simulink model "vloop_test_modify2017"  (R2017a)
settings: Solver=FixedStepAuto  StartTime=0.0  StopTime=Tf  FixedStep=delta_r  RelTol=1e-3  EnableMultiTasking=on
InitFcn:
  | G = 107.815;
values from neighbouring files (symbols this model uses):
  delta_r = 1/1000    (= 0.001)    [p560_simulation_main_velocity2017.m]
  delta_t = 1/200    (= 0.005)    [p560_simulation_main_velocity2017.m]
  Kd = 0.0006    [p560_simulation_main_velocity2017.m]
  time_delay = 0    [p560_simulation_main_velocity2017.m]
undefined symbols (not defined in the file or in its folder): yh
libraries: sldrtlib x1, simulink x1
Description:
  | vloop parameters for
  | Puma560 shoulder joint
  | with link inertia
  | RVC1 p.205
settings Model: DisableUpgradeWarningsForVersion=R2014b  Creator=pic  LastModifiedBy=yehanspc
settings DataIOCC: LimitDataPoints=on  SaveFormat=Array  SignalLoggingSaveFormat=ModelDataLogs  ReturnWorkspaceOutputs=on  TimeSaveName=t  OutputSaveName=y
settings OptimizationCC: ExpressionDepthLimit=2147483647  LifeSpan=inf
settings DebuggingCC: UnderspecifiedInitializationDetection=Classic  MergeDetectMultiDrivingBlocksExec=none  SolverPrmCheckMsg=warning  MultiTaskRateTransMsg=warning  FcnCallInpInsideContextMsg=warning  AllowSymbolicDim=off  StateNameClashWarn=warning  SFUnexpectedBacktrackingDiag=warning  SFNoUnconditionalDefaultTransitionDiag=warning  SFExecutionAtInitializationDiag=none
settings HardwareCC: ProdBitPerPointer=32  ProdBitPerSizeT=32  ProdBitPerPtrDiffT=32  ProdLargestAtomicFloat=None  ProdIntDivRoundTo=Undefined  ProdEndianess=Unspecified  ProdWordSize=32  ProdHWDeviceType=32-bit Generic
settings ModelReferenceCC: PropagateSignalLabelsOutOfModel=off
settings SFSimCC: SimCustomInitializer=|
  | if ~exist(tau_d)
  |    tau_d = 0
  | end
settings GRTTargetCC: TargetLangStandard=C89/C90 (ANSI)  GeneratePreprocessorConditionals=Disable all  CombineOutputUpdateFcns=off  GRTInterface=on
settings ConfigComp: CovMetricSettings=dw  CovHtmlReporting=on  CovSaveCumulativeToWorkspaceVar=on  CovSaveSingleToWorkspaceVar=on  CovExternalEMLEnable=off  CovSFcnEnable=off

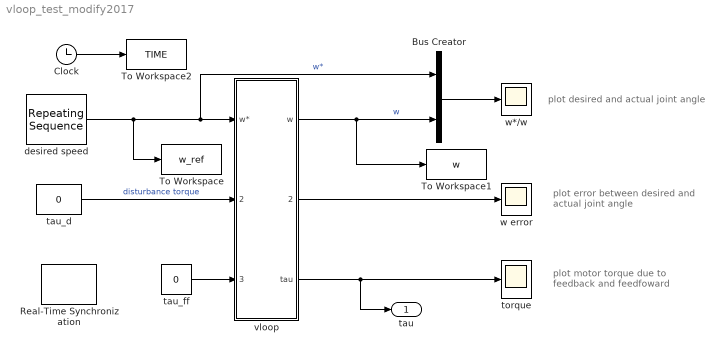
== system vloop_test_modify2017 ==
  note: plot motor torque due
      | to feedback and feedfoward
  note: plot error between desired and
      | actual joint angle
  note: plot desired and actual joint angle
  Bus Creator : BusCreator  Inputs=2
  Clock : Clock
  Real-Time Synchronization : sldrtlib/Real-Time Synchronization  SampleTime=delta_t  MaxMissedTicks=10000  ShowMissedTicks=off  YieldWhenWaiting=off
  To Workspace : ToWorkspace  VariableName=w_ref  SaveFormat=Timeseries  SampleTime=-1
  To Workspace1 : ToWorkspace  VariableName=w  SaveFormat=Timeseries  SampleTime=-1
  To Workspace2 : ToWorkspace  VariableName=TIME  SaveFormat=Timeseries  SampleTime=-1
  desired speed : simulink/Sources/Repeating Sequence  rep_seq_t=[0 1 3 4 6]/10  rep_seq_y=[50 50 50 50 50]
  tau_d : Constant  Value=0
  tau_ff : Constant  Value=0
  torque : Scope
  vloop : Subsystem  AncestorBlock=roblocks/Arm/vloop  mask{J=580e-6, B=817e-6, Km=0.228, tau_max=0.9, Kv=0.3, Ki=0.2, T=0.001}
      mask prompts: J "Inertia (J)"; B "Viscous friction coefficient (B)"; Km "Motor torque constant"; tau_max "Torque limit (tau_max)"; Kv "Proportional gain (Kv)"; Ki "Integral gain (Ki)"; T "Sample interval (T)"
  w error : Scope
  w*/w : Scope
  tau : Outport
  wires:
  desired speed/1 -> To Workspace/1, Bus Creator/1, vloop/1(w*)  "w*"
  Bus Creator/1 -> w*/w/1
  vloop/1(w) -> To Workspace1/1, Bus Creator/2  "w"
  vloop/2(w error) -> w error/1
  vloop/3(tau) -> torque/1, tau/1
  tau_d/1 -> vloop/2(tau_d)  "disturbance torque"
  tau_ff/1 -> vloop/3(tau_ff)
  Clock/1 -> To Workspace2/1

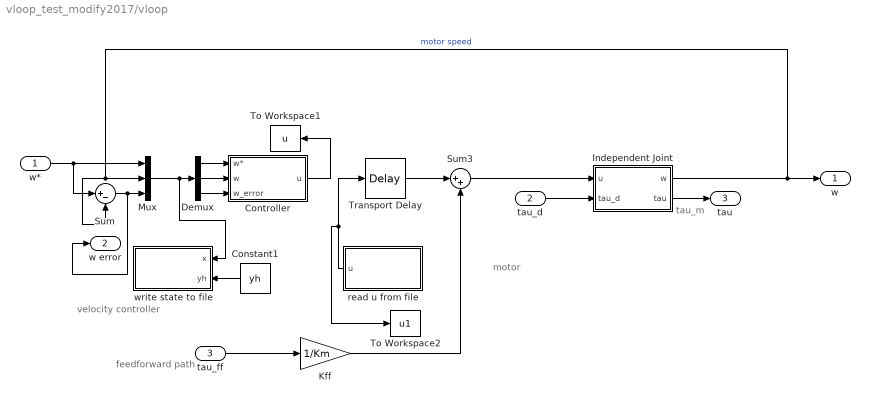
== system vloop_test_modify2017/vloop ==
  note: velocity controller
  note: feedforward path
  note: tau_m
  note: motor
  w* : Inport
  tau_d : Inport  Port=2
  tau_ff : Inport  Port=3
  Constant1 : Constant  Value=yh
  Controller : Subsystem
  Demux : Demux  Outputs=3
  Independent Joint : Subsystem
  Kff : Gain  Gain=1/Km
  Mux : Mux  Inputs=3
  Sum : Sum  Inputs=|+-
  Sum3 : Sum  Inputs=|++
  To Workspace1 : ToWorkspace  VariableName=u  SaveFormat=Timeseries  SampleTime=-1
  To Workspace2 : ToWorkspace  VariableName=u1  SaveFormat=Timeseries  SampleTime=-1
  Transport Delay : TransportDelay  DelayTime=time_delay
  read u from file : MATLAB Function  TreatAsAtomicUnit=on
  write state to file : MATLAB Function  TreatAsAtomicUnit=on
  w : Outport
  w error : Outport  Port=2
  tau : Outport  Port=3
  wires:
  tau_ff/1 -> Kff/1
  Kff/1 -> Sum3/2
  Sum3/1 -> Independent Joint/1(u)
  tau_d/1 -> Independent Joint/2(tau_d)
  Independent Joint/1(w) -> Mux/2, Sum/2, w/1  "motor speed"
  w*/1 -> Mux/1, Sum/1
  Sum/1 -> Mux/3, w error/1
  Transport Delay/1 -> Sum3/1
  Independent Joint/2(tau) -> tau/1
  Mux/1 -> Demux/1, write state to file/1(x)
  Constant1/1 -> write state to file/2(yh)
  Demux/1 -> Controller/1(w*)
  Demux/2 -> Controller/2(w)
  Demux/3 -> Controller/3(w_error)
  Controller/1(u) -> To Workspace1/1
  read u from file/1(u) -> To Workspace2/1, Transport Delay/1

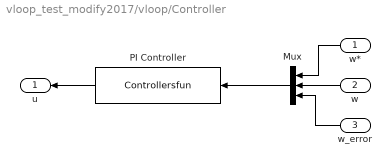
== system vloop_test_modify2017/vloop/Controller ==
  w* : Inport
  w : Inport  Port=2
  w_error : Inport  Port=3
  Mux : Mux  Inputs=3
  PI Controller : S-Function  FunctionName=Controllersfun  Parameters=Kv,Ki,Kd,delta_t,delta_r  SFunctionDeploymentMode=off  EnableBusSupport=off
  u : Outport
  wires:
  w/1 -> Mux/2
  w*/1 -> Mux/1
  Mux/1 -> PI Controller/1
  PI Controller/1 -> u/1
  w_error/1 -> Mux/3

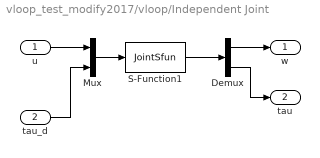
== system vloop_test_modify2017/vloop/Independent Joint ==
  u : Inport
  tau_d : Inport  Port=2
  Demux : Demux  Outputs=2
  Mux : Mux  Inputs=2
  S-Function1 : S-Function  FunctionName=JointSfun  Parameters=B,J,Km,delta_r  SFunctionDeploymentMode=off  EnableBusSupport=off
  w : Outport
  tau : Outport  Port=2
  wires:
  Mux/1 -> S-Function1/1
  u/1 -> Mux/1
  tau_d/1 -> Mux/2
  S-Function1/1 -> Demux/1
  Demux/1 -> w/1
  Demux/2 -> tau/1

== matlab function vloop_test_modify2017/vloop/write state to file ==
  data: x input; yh input
function write_block(x,yh)
% Inputs:
% ymea: measurement from structure
% Outputs:
% ymea1: measurement output

eml.extrinsic('write_x');
write_x(x,yh);

== matlab function vloop_test_modify2017/vloop/read u from file ==
  data: u output
function u = read_u_block
% Inputs:
% ymea: measurement from structure
% Outputs:
% ymea1: measurement output

% coder.extrinsic('fscanf')
u=0;
eml.extrinsic('read_u');
% 
u = read_u();
